simulink model "Rodriguez20213058 [Simulink abierto]"  (R2024b)
settings: Solver=ode15s  StartTime=1E-3  StopTime=10  MaxStep=1E-3  RelTol=1e-3
settings Model: Creator=mluser
settings DataIOCC: ReturnWorkspaceOutputs=off  TimeSaveName=t
settings DebuggingCC: AlgebraicLoopMsg=none  InheritedTsInSrcMsg=none
settings RTWCC: GPUComputeCapability=3.5

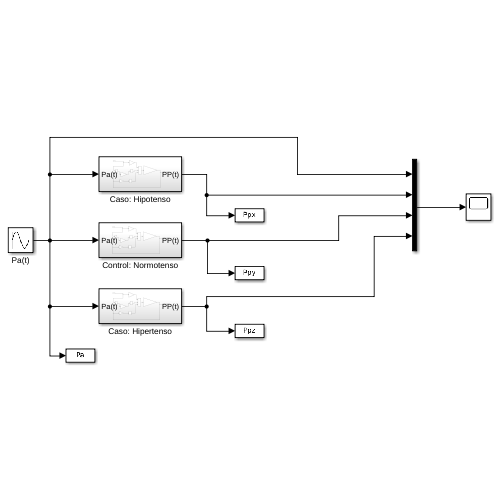
[thumbnail: Simulink's stored preview of the top-level diagram]
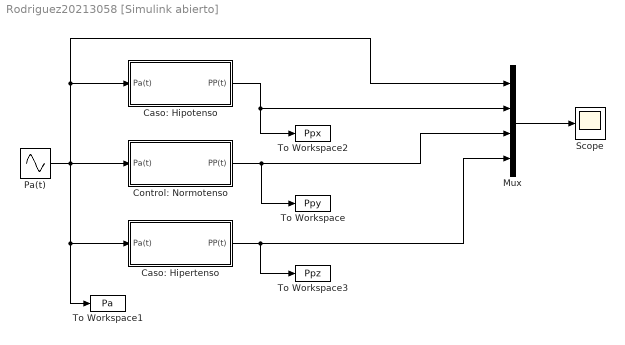
== system Rodriguez20213058 [Simulink abierto] ==
  Caso: Hipertenso : Subsystem
  Caso: Hipotenso : Subsystem
  Control: Normotenso : Subsystem
  Mux : Mux
  Pa(t) : Sin  Bias=0.8  Frequency=9.42
  Scope : Scope
  To Workspace : ToWorkspace  VariableName=Ppy  SampleTime=-1
  To Workspace1 : ToWorkspace  VariableName=Pa  SampleTime=-1
  To Workspace2 : ToWorkspace  VariableName=Ppx  SampleTime=-1
  To Workspace3 : ToWorkspace  VariableName=Ppz  SampleTime=-1
  wires:
  Mux/1 -> Scope/1
  Pa(t)/1 -> Control: Normotenso/1(Pa(t)), Caso: Hipotenso/1(Pa(t)), Mux/1, Caso: Hipertenso/1(Pa(t)), To Workspace1/1
  Control: Normotenso/1(PP(t)) -> To Workspace/1, Mux/3
  Caso: Hipotenso/1(PP(t)) -> To Workspace2/1, Mux/2
  Caso: Hipertenso/1(PP(t)) -> To Workspace3/1, Mux/4

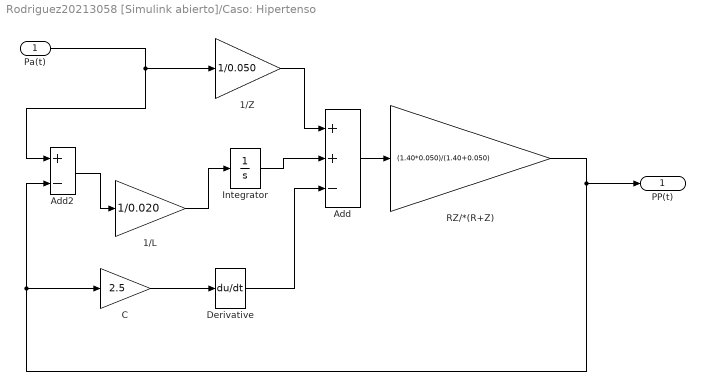
== system Rodriguez20213058 [Simulink abierto]/Caso: Hipertenso ==
  Pa(t) : Inport
  1/L : Gain  Gain=1/0.020
  1/Z : Gain  Gain=1/0.050
  Add : Sum  Inputs=++-
  Add2 : Sum  Inputs=+-
  C : Gain  Gain=2.5
  Derivative : Derivative
  Integrator : Integrator
  RZ/*(R+Z) : Gain  Gain=(1.40*0.050)/(1.40+0.050)
  PP(t) : Outport
  wires:
  Add/1 -> RZ/*(R+Z)/1
  Pa(t)/1 -> Add2/1, 1/Z/1
  1/Z/1 -> Add/1
  1/L/1 -> Integrator/1
  Add2/1 -> 1/L/1
  C/1 -> Derivative/1
  RZ/*(R+Z)/1 -> C/1, Add2/2, PP(t)/1
  Derivative/1 -> Add/3
  Integrator/1 -> Add/2

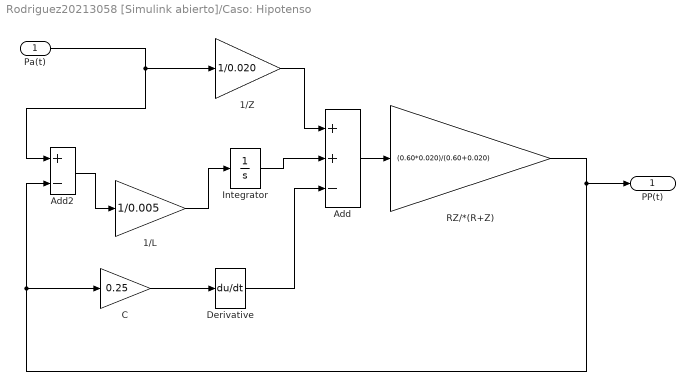
== system Rodriguez20213058 [Simulink abierto]/Caso: Hipotenso ==
  Pa(t) : Inport
  1/L : Gain  Gain=1/0.005
  1/Z : Gain  Gain=1/0.020
  Add : Sum  Inputs=++-
  Add2 : Sum  Inputs=+-
  C : Gain  Gain=0.25
  Derivative : Derivative
  Integrator : Integrator
  RZ/*(R+Z) : Gain  Gain=(0.60*0.020)/(0.60+0.020)
  PP(t) : Outport
  wires:
  C/1 -> Derivative/1
  Add/1 -> RZ/*(R+Z)/1
  Add2/1 -> 1/L/1
  1/Z/1 -> Add/1
  Integrator/1 -> Add/2
  1/L/1 -> Integrator/1
  RZ/*(R+Z)/1 -> C/1, Add2/2, PP(t)/1
  Pa(t)/1 -> Add2/1, 1/Z/1
  Derivative/1 -> Add/3

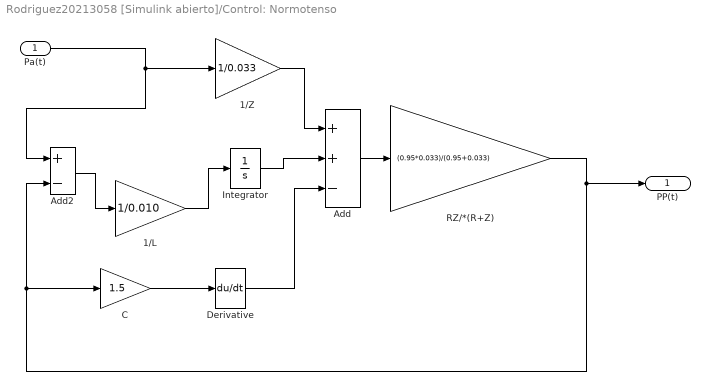
== system Rodriguez20213058 [Simulink abierto]/Control: Normotenso ==
  Pa(t) : Inport
  1/L : Gain  Gain=1/0.010
  1/Z : Gain  Gain=1/0.033
  Add : Sum  Inputs=++-
  Add2 : Sum  Inputs=+-
  C : Gain  Gain=1.5
  Derivative : Derivative
  Integrator : Integrator
  RZ/*(R+Z) : Gain  Gain=(0.95*0.033)/(0.95+0.033)
  PP(t) : Outport
  wires:
  C/1 -> Derivative/1
  Add2/1 -> 1/L/1
  1/Z/1 -> Add/1
  RZ/*(R+Z)/1 -> C/1, Add2/2, PP(t)/1
  Add/1 -> RZ/*(R+Z)/1
  1/L/1 -> Integrator/1
  Pa(t)/1 -> Add2/1, 1/Z/1
  Integrator/1 -> Add/2
  Derivative/1 -> Add/3
